simulink model "QEM"  (R2019b)
settings: Solver=VariableStepAuto  StartTime=0.0  StopTime=10.0  RelTol=1e-3
libraries: arduinolib x1
settings Model: Creator=dell  LastModifiedBy=covasanvictor
settings DataIOCC: ReturnWorkspaceOutputs=off
settings DebuggingCC: ArithmeticOperatorsInVariantConditions=warning
settings SFSimCC: CustomCodeUndefinedFunction=UseInterfaceOnly

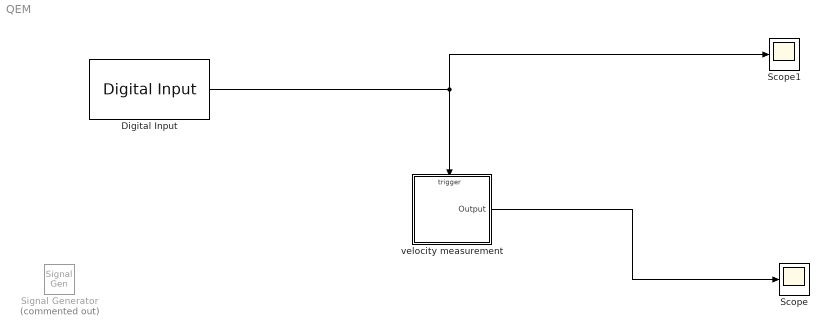
== system QEM ==
  Digital Input : arduinolib/Digital Input  pinNumber=8  SampleTime=0.1  blockPlatform=arduino
      settings: SourceProductName=Simulink Support Package for Arduino Hardware
  Scope : Scope
  Scope1 : Scope
  Signal Generator : SignalGenerator  Commented=on  Units=rad/sec
  "velocity measurement " : Subsystem
  wires:
  "velocity measurement "/1(Output) -> Scope/1
  Digital Input/1 -> Scope1/1, "velocity measurement "/Trigger

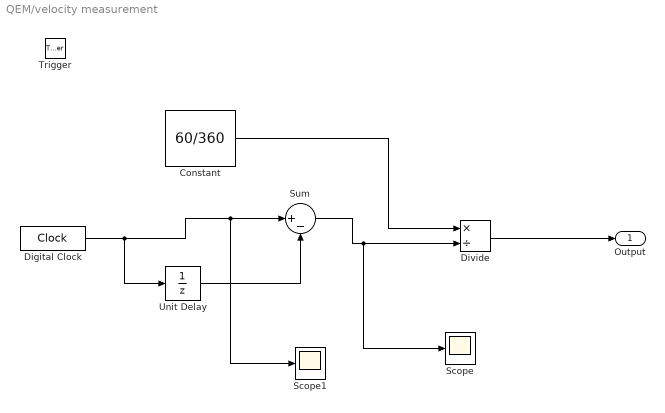
== system QEM/velocity measurement  ==
  Trigger : TriggerPort  TriggerType=either  VariantControl=Variant  OutputDataType=double  PortDimensions=1
  Constant : Constant  Value=60/360  SampleTime=-1
  Digital Clock : DigitalClock  SampleTime=-1
  Divide : Product  Inputs=*/
  Scope : Scope
  Scope1 : Scope
  Sum : Sum  Inputs=|+-
  Unit Delay : UnitDelay  SampleTime=-1  HasFrameUpgradeWarning=on
  Output : Outport  VectorParamsAs1DForOutWhenUnconnected=off
  wires:
  Unit Delay/1 -> Sum/2
  Digital Clock/1 -> Unit Delay/1, Scope1/1, Sum/1
  Divide/1 -> Output/1
  Constant/1 -> Divide/1
  Sum/1 -> Scope/1, Divide/2
